simulink model "orig"  (R2018a)
settings: Solver=VariableStepAuto  StartTime=0.0  StopTime=10.0  RelTol=1e-3
undefined symbols (not defined in the file): DiscIntNeverNeededParam
libraries: simulink x6
settings Model: Creator=ishaf  LastModifiedBy=ishaf

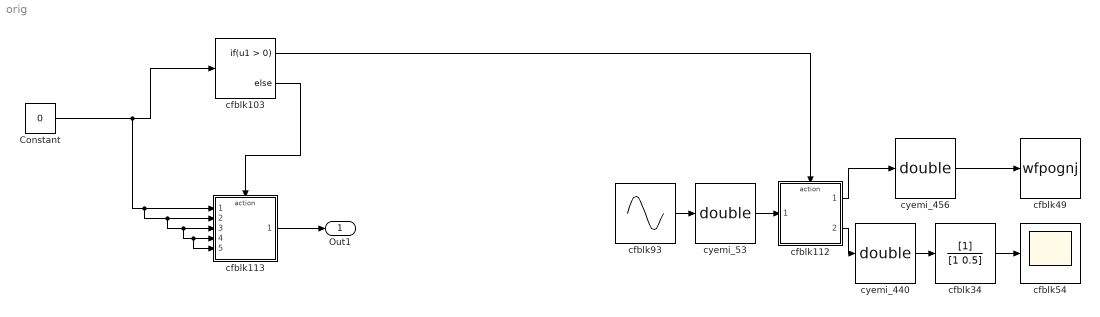
== system orig ==
  Constant : Constant  Value=0
  cfblk103 : If  SampleTime=1
  cfblk112 : Subsystem  TreatAsAtomicUnit=on
  cfblk113 : Subsystem  TreatAsAtomicUnit=on
  cfblk34 : DiscreteFilter  SampleTime=1
  cfblk49 : ToWorkspace  VariableName=wfpognj  SaveFormat=Timeseries  SampleTime=-1
  cfblk54 : Scope
  cfblk93 : Sin  SampleTime=0
  cyemi_440 : DataTypeConversion  OutDataTypeStr=double
  cyemi_456 : DataTypeConversion  OutDataTypeStr=double
  cyemi_53 : DataTypeConversion  OutDataTypeStr=double
  Out1 : Outport
  wires:
  cyemi_53/1 -> cfblk112/1(cfblk1)
  cfblk112/1(cfblk2) -> cyemi_456/1
  cfblk112/2(cfblk9) -> cyemi_440/1
  cfblk93/1 -> cyemi_53/1
  cyemi_456/1 -> cfblk49/1
  cfblk34/1 -> cfblk54/1
  cyemi_440/1 -> cfblk34/1
  Constant/1 -> cfblk113/5(cfblk15), cfblk113/4(cfblk14), cfblk113/3(cfblk13), cfblk113/2(cfblk12), cfblk113/1(cfblk1), cfblk103/1
  cfblk103/1 -> cfblk112/Action
  cfblk103/2 -> cfblk113/Action
  cfblk113/1(cfblk2) -> Out1/1

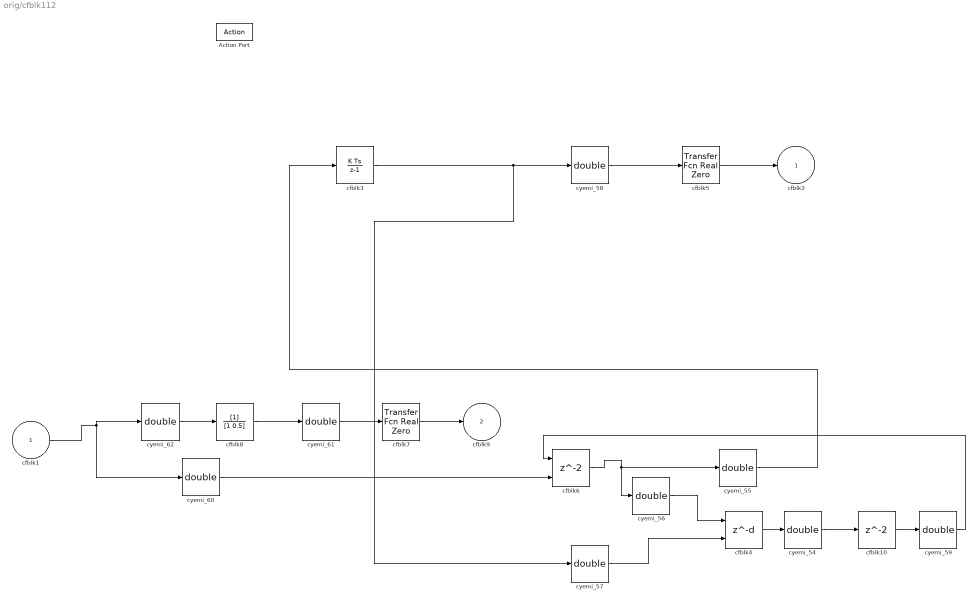
== system orig/cfblk112 ==
  cfblk1 : Inport
  Action Port : ActionPort  ActionType=then
  cfblk10 : Delay
  cfblk3 : DiscreteIntegrator  SampleTime=-1  OutDataTypeStr=double  ICPrevOutput=DiscIntNeverNeededParam  ICPrevScaledInput=DiscIntNeverNeededParam
  cfblk4 : Delay  DelayLengthSource=Input port
      settings: InputPortMap=u0,p1
  cfblk5 : simulink/Discrete/Transfer Fcn Real Zero  ZeroZ=0.75  ICPrevInput=0.0  DoSatur=off
      settings: SourceProductName=Simulink  SourceProductBaseCode=SL
  cfblk6 : Delay  ShowEnablePort=on
      settings: InputPortMap=u0,e6
  cfblk7 : simulink/Discrete/Transfer Fcn Real Zero  ZeroZ=0.75  ICPrevInput=0.0  DoSatur=off
      settings: SourceProductName=Simulink  SourceProductBaseCode=SL
  cfblk8 : DiscreteFilter
  cyemi_{54..62} (9 alike) : DataTypeConversion  OutDataTypeStr=double
  cfblk2 : Outport
  cfblk9 : Outport  Port=2
  wires:
  cfblk6/1 -> cyemi_56/1, cyemi_55/1
  cfblk7/1 -> cfblk9/1
  cfblk3/1 -> cyemi_57/1, cyemi_58/1
  cfblk1/1 -> cyemi_62/1, cyemi_60/1
  cfblk5/1 -> cfblk2/1
  cyemi_54/1 -> cfblk10/1
  cfblk4/1 -> cyemi_54/1
  cyemi_55/1 -> cfblk3/1
  cyemi_56/1 -> cfblk4/1
  cyemi_57/1 -> cfblk4/2
  cyemi_58/1 -> cfblk5/1
  cyemi_59/1 -> cfblk6/1
  cfblk10/1 -> cyemi_59/1
  cyemi_60/1 -> cfblk6/2
  cyemi_61/1 -> cfblk7/1
  cfblk8/1 -> cyemi_61/1
  cyemi_62/1 -> cfblk8/1

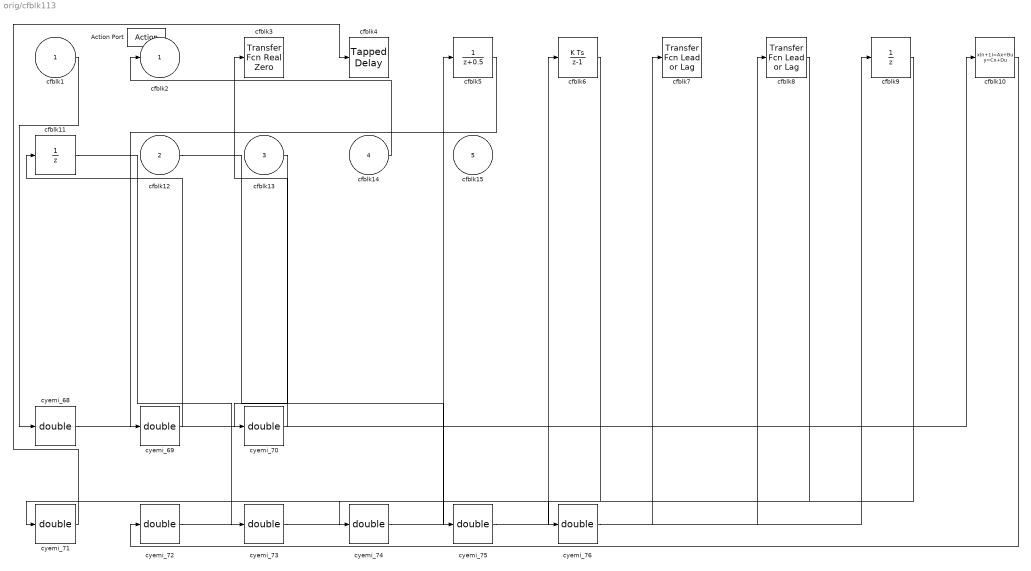
== system orig/cfblk113 ==
  cfblk1 : Inport
  cfblk12 : Inport  Port=2
  cfblk13 : Inport  Port=3
  cfblk14 : Inport  Port=4
  cfblk15 : Inport  Port=5
  Action Port : ActionPort  ActionType=else
  cfblk10 : DiscreteStateSpace  SampleTime=-1
  cfblk11 : UnitDelay  SampleTime=-1
  cfblk3 : simulink/Discrete/Transfer Fcn Real Zero  ZeroZ=0.75  ICPrevInput=0.0  DoSatur=off
      settings: SourceProductName=Simulink  SourceProductBaseCode=SL
  cfblk4 : simulink/Discrete/Tapped Delay  vinit=0.0  samptime=-1  NumDelays=1  DelayOrder=Oldest  includeCurrent=off
  cfblk5 : DiscreteTransferFcn
  cfblk6 : DiscreteIntegrator  SampleTime=-1  OutDataTypeStr=double  ICPrevOutput=DiscIntNeverNeededParam  ICPrevScaledInput=DiscIntNeverNeededParam
  cfblk7 : simulink/Discrete/Transfer Fcn Lead or Lag  PoleZ=0.95  ZeroZ=0.75  ICPrevOutput=0.0  ICPrevInput=0.0  DoSatur=off
      settings: SourceProductName=Simulink  SourceProductBaseCode=SL
  cfblk8 : simulink/Discrete/Transfer Fcn Lead or Lag  PoleZ=0.95  ZeroZ=0.75  ICPrevOutput=0.0  ICPrevInput=0.0  DoSatur=off
      settings: SourceProductName=Simulink  SourceProductBaseCode=SL
  cfblk9 : UnitDelay  SampleTime=-1
  cyemi_{68..76} (9 alike) : DataTypeConversion  OutDataTypeStr=double
  cfblk2 : Outport
  wires:
  cfblk14/1 -> cfblk2/1
  cyemi_68/1 -> cfblk10/1
  cfblk1/1 -> cyemi_68/1
  cyemi_69/1 -> cfblk11/1
  cfblk5/1 -> cyemi_69/1
  cyemi_70/1 -> cfblk3/1
  cfblk13/1 -> cyemi_70/1
  cyemi_71/1 -> cfblk4/1
  cfblk9/1 -> cyemi_71/1
  cyemi_72/1 -> cfblk5/1
  cfblk10/1 -> cyemi_72/1
  cyemi_73/1 -> cfblk6/1
  cfblk11/1 -> cyemi_73/1
  cyemi_74/1 -> cfblk7/1
  cfblk8/1 -> cyemi_74/1
  cyemi_75/1 -> cfblk8/1
  cfblk12/1 -> cyemi_75/1
  cyemi_76/1 -> cfblk9/1
  cfblk6/1 -> cyemi_76/1
